simulink model "before_MPC"  (R2022b)
settings: Solver=VariableStepAuto  StartTime=0.0  StopTime=1e6  RelTol=1e-3
values from neighbouring files (symbols this model uses):
  BC = m/A/Cd    (= 136.363636364)    [ARES.m]    (also in control_before_MPC.m = 122; reference_signal_291123.m = 122; validation.m)
  Cd = 2.2    [ARES.m]    (also in control_before_MPC.m; control_script_291123.m; reference_signal_291123.m; validation.m)
  CL = Cd*E    (= 0)    [ARES.m]    (also in control_before_MPC.m; control_script_291123.m; reference_signal_291123.m; validation.m)
  F107_avg = 90.85    [ARES.m]    (also in control_before_MPC.m; control_script_291123.m; reference_signal_291123.m; validation.m)
  F107_day = 86.0    (= 86)    [ARES.m]    (also in control_before_MPC.m; control_script_291123.m; reference_signal_291123.m; validation.m)
  gamma0 = kepOut.gamma(end)    [ARES.m]    (also in control_before_MPC.m; control_script_291123.m; reference_signal_291123.m; validation.m)
  h0 = kepOut.h(end)    [ARES.m]    (also in control_before_MPC.m; control_script_291123.m; getSH.m = h0(n); reference_signal_291123.m)
  jdate = jdate+ndays1    [ARES.m]    (also in control_before_MPC.m; control_script_291123.m; reference_signal_291123.m; validation.m)
  Kp = 1    [ARES.m]    (also in control_before_MPC.m; control_script_291123.m; reference_signal_291123.m; validation.m)
  mi = 398600.44    [ARES.m]    (also in control_before_MPC.m; control_script_291123.m; reference_signal_291123.m; validation.m)
  r_a = alt_0+Re    (= 6771.0088)    [ARES.m]    (also in control_before_MPC.m = 6571.0088; control_script_291123.m = 6571.0088; reference_signal_291123.m = 6571.0088; validation.m = 6571.0088)
  Re = Re*1000    (= 6371008.8)    [ARES.m]    (also in control_before_MPC.m; control_script_291123.m; reference_signal_291123.m; trajectory_solver.m = 6378000)
  stop_h = 0    [ARES.m]    (also in control_before_MPC.m; control_script_291123.m; reference_signal_291123.m; validation.m)
  theta0 = kepOut.theta(end)    [ARES.m]    (also in control_before_MPC.m; control_script_291123.m; reference_signal_291123.m; validation.m)
  V0 = kepOut.V(end)    [ARES.m]    (also in control_before_MPC.m; control_script_291123.m; reference_signal_291123.m; validation.m)
  x0 = kepOut.x(end)    [ARES.m]    (also in control_before_MPC.m; control_script_291123.m; reference_signal_291123.m; validation.m)
libraries: simulink x2
settings Model: Creator=zhanghanwen  LastModifiedBy=zhanghanwen

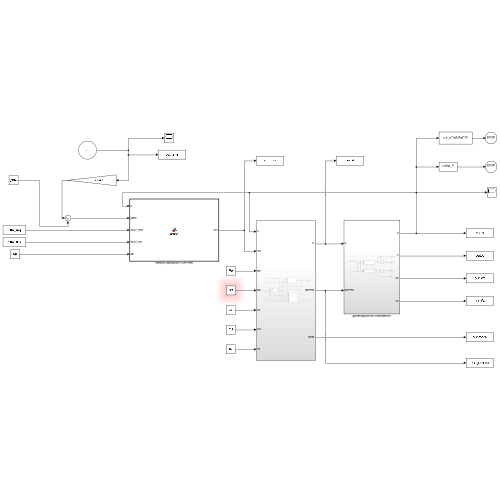
[thumbnail: Simulink's stored preview of the top-level diagram]
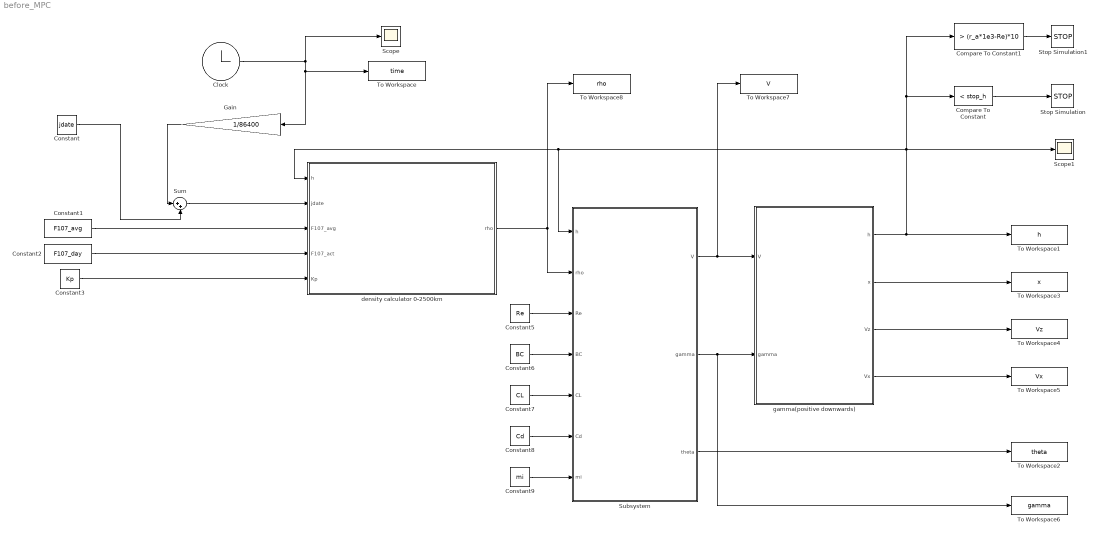
== system before_MPC ==
  Clock : Clock
  Compare To Constant : simulink/Logic and Bit Operations/Compare To Constant  relop=<  const=stop_h  OutDataTypeStr=boolean
  Compare To Constant1 : simulink/Logic and Bit Operations/Compare To Constant  relop=>  const=(r_a*1e3-Re)*10  OutDataTypeStr=boolean
  Constant : Constant  Value=jdate
  Constant1 : Constant  Value=F107_avg
  Constant2 : Constant  Value=F107_day
  Constant3 : Constant  Value=Kp
  Constant5 : Constant  Value=Re
  Constant6 : Constant  Value=BC
  Constant7 : Constant  Value=CL
  Constant8 : Constant  Value=Cd
  Constant9 : Constant  Value=mi
  Gain : Gain  Gain=1/86400
  Scope : Scope
  Scope1 : Scope
  Stop Simulation : Stop
  Stop Simulation1 : Stop
  Subsystem : Subsystem
  Sum : Sum  Inputs=|++
  To Workspace : ToWorkspace  VariableName=time  SampleTime=-1
      settings: Save2DSignal=2-D array (concatenate along first dimension)
  To Workspace1 : ToWorkspace  VariableName=h  SampleTime=-1
      settings: Save2DSignal=2-D array (concatenate along first dimension)
  To Workspace2 : ToWorkspace  VariableName=theta  SampleTime=-1
      settings: Save2DSignal=2-D array (concatenate along first dimension)
  To Workspace3 : ToWorkspace  VariableName=x  SampleTime=-1
  To Workspace4 : ToWorkspace  VariableName=Vz  SampleTime=-1
      settings: Save2DSignal=2-D array (concatenate along first dimension)
  To Workspace5 : ToWorkspace  VariableName=Vx  SampleTime=-1
      settings: Save2DSignal=2-D array (concatenate along first dimension)
  To Workspace6 : ToWorkspace  VariableName=gamma  SampleTime=-1
      settings: Save2DSignal=2-D array (concatenate along first dimension)
  To Workspace7 : ToWorkspace  VariableName=V  SampleTime=-1
      settings: Save2DSignal=2-D array (concatenate along first dimension)
  To Workspace8 : ToWorkspace  VariableName=rho  SampleTime=-1
      settings: Save2DSignal=2-D array (concatenate along first dimension)
  density calculator 0-2500km : MATLAB Function  TreatAsAtomicUnit=on
  gamma(positive downwards) : Subsystem
  wires:
  Clock/1 -> Gain/1, To Workspace/1, Scope/1
  Constant/1 -> Sum/2
  Sum/1 -> density calculator 0-2500km/2(jdate)
  Constant1/1 -> density calculator 0-2500km/3(F107_avg)
  Constant2/1 -> density calculator 0-2500km/4(F107_act)
  Constant3/1 -> density calculator 0-2500km/5(Kp)
  Gain/1 -> Sum/1
  density calculator 0-2500km/1(rho) -> To Workspace8/1, Subsystem/2(rho)
  Constant5/1 -> Subsystem/3(Re)
  Constant6/1 -> Subsystem/4(BC)
  Constant7/1 -> Subsystem/5(CL)
  Constant8/1 -> Subsystem/6(Cd)
  Constant9/1 -> Subsystem/7(mi)
  Subsystem/3(theta) -> To Workspace2/1
  Subsystem/2(gamma) -> To Workspace6/1, gamma(positive downwards)/2(gamma)
  Subsystem/1(V) -> To Workspace7/1, gamma(positive downwards)/1(V)
  gamma(positive downwards)/2(x) -> To Workspace3/1
  gamma(positive downwards)/3(Vz) -> To Workspace4/1
  gamma(positive downwards)/4(Vx) -> To Workspace5/1
  gamma(positive downwards)/1(h) -> Compare To Constant1/1, Compare To Constant/1, Subsystem/1(h), density calculator 0-2500km/1(h), Scope1/1, To Workspace1/1
  Compare To Constant/1 -> Stop Simulation/1
  Compare To Constant1/1 -> Stop Simulation1/1

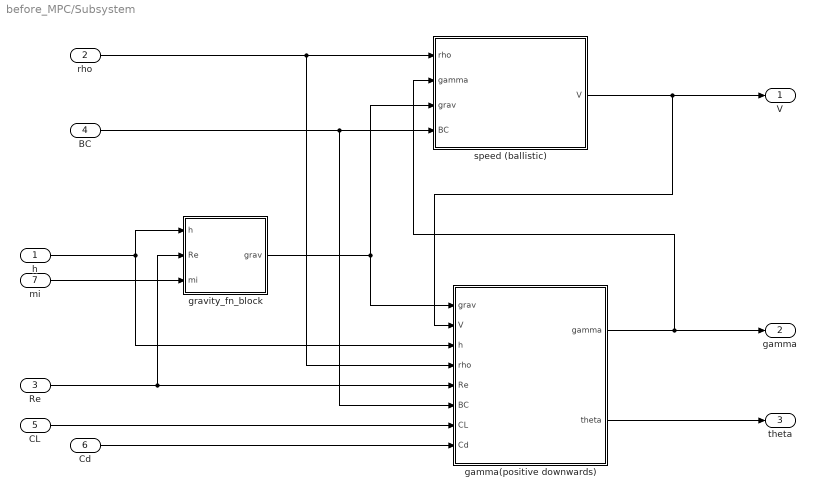
== system before_MPC/Subsystem ==
  h : Inport
  rho : Inport  Port=2
  Re : Inport  Port=3
  BC : Inport  Port=4
  CL : Inport  Port=5
  Cd : Inport  Port=6
  mi : Inport  Port=7
  gamma(positive downwards) : Subsystem
  gravity_fn_block : MATLAB Function  TreatAsAtomicUnit=on
  speed (ballistic) : Subsystem
  V : Outport
  gamma : Outport  Port=2
  theta : Outport  Port=3
  wires:
  rho/1 -> gamma(positive downwards)/4(rho), speed (ballistic)/1(rho)
  gravity_fn_block/1(grav) -> speed (ballistic)/3(grav), gamma(positive downwards)/1(grav)
  h/1 -> gravity_fn_block/1(h), gamma(positive downwards)/3(h)
  gamma(positive downwards)/1(gamma) -> speed (ballistic)/2(gamma), gamma/1
  gamma(positive downwards)/2(theta) -> theta/1
  speed (ballistic)/1(V) -> V/1, gamma(positive downwards)/2(V)
  Re/1 -> gravity_fn_block/2(Re), gamma(positive downwards)/5(Re)
  BC/1 -> gamma(positive downwards)/6(BC), speed (ballistic)/4(BC)
  CL/1 -> gamma(positive downwards)/7(CL)
  Cd/1 -> gamma(positive downwards)/8(Cd)
  mi/1 -> gravity_fn_block/3(mi)

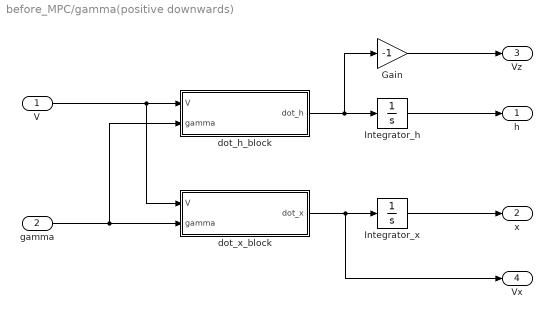
== system before_MPC/gamma(positive downwards) ==
  V : Inport
  gamma : Inport  Port=2
  Gain : Gain  Gain=-1
  Integrator_h : Integrator  InitialCondition=h0
  Integrator_x : Integrator  InitialCondition=x0
  dot_h_block : MATLAB Function  TreatAsAtomicUnit=on
  dot_x_block : MATLAB Function  TreatAsAtomicUnit=on
  h : Outport
  x : Outport  Port=2
  Vz : Outport  Port=3
  Vx : Outport  Port=4
  wires:
  V/1 -> dot_x_block/1(V), dot_h_block/1(V)
  gamma/1 -> dot_x_block/2(gamma), dot_h_block/2(gamma)
  Integrator_h/1 -> h/1
  dot_h_block/1(dot_h) -> Gain/1, Integrator_h/1
  Integrator_x/1 -> x/1
  dot_x_block/1(dot_x) -> Vx/1, Integrator_x/1
  Gain/1 -> Vz/1

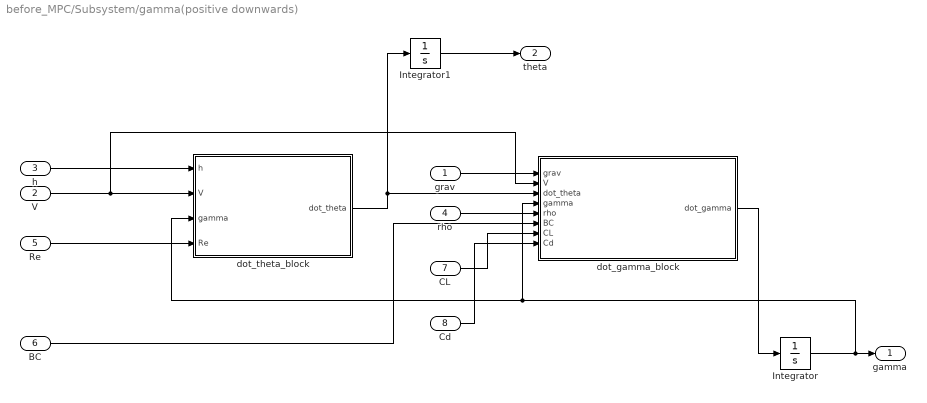
== system before_MPC/Subsystem/gamma(positive downwards) ==
  grav : Inport
  V : Inport  Port=2
  h : Inport  Port=3
  rho : Inport  Port=4
  Re : Inport  Port=5
  BC : Inport  Port=6
  CL : Inport  Port=7
  Cd : Inport  Port=8
  Integrator : Integrator  InitialCondition=gamma0  AbsoluteTolerance=1e-6  ZeroCross=off
  Integrator1 : Integrator  InitialCondition=theta0
  dot_gamma_block : MATLAB Function  TreatAsAtomicUnit=on
  dot_theta_block : MATLAB Function  TreatAsAtomicUnit=on
  gamma : Outport
  theta : Outport  Port=2
  wires:
  grav/1 -> dot_gamma_block/1(grav)
  dot_gamma_block/1(dot_gamma) -> Integrator/1
  dot_theta_block/1(dot_theta) -> Integrator1/1, dot_gamma_block/3(dot_theta)
  rho/1 -> dot_gamma_block/5(rho)
  h/1 -> dot_theta_block/1(h)
  V/1 -> dot_gamma_block/2(V), dot_theta_block/2(V)
  Integrator1/1 -> theta/1
  Integrator/1 -> dot_theta_block/3(gamma), dot_gamma_block/4(gamma), gamma/1
  Re/1 -> dot_theta_block/4(Re)
  BC/1 -> dot_gamma_block/6(BC)
  CL/1 -> dot_gamma_block/7(CL)
  Cd/1 -> dot_gamma_block/8(Cd)

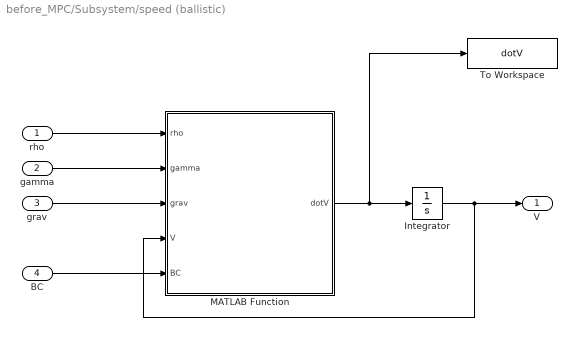
== system before_MPC/Subsystem/speed (ballistic) ==
  rho : Inport
  gamma : Inport  Port=2
  grav : Inport  Port=3
  BC : Inport  Port=4
  Integrator : Integrator  InitialCondition=V0
  MATLAB Function : MATLAB Function  TreatAsAtomicUnit=on
  To Workspace : ToWorkspace  VariableName=dotV  SampleTime=-1
      settings: Save2DSignal=2-D array (concatenate along first dimension)
  V : Outport
  wires:
  Integrator/1 -> MATLAB Function/4(V), V/1
  grav/1 -> MATLAB Function/3(grav)
  gamma/1 -> MATLAB Function/2(gamma)
  rho/1 -> MATLAB Function/1(rho)
  MATLAB Function/1(dotV) -> Integrator/1, To Workspace/1
  BC/1 -> MATLAB Function/5(BC)

== matlab function before_MPC/Subsystem/gravity_fn_block ==
  data: h input; grav output; Re input; mi input
function grav = gravity(h,Re,mi)

grav = mi*1e9 / (Re+h)^2;
end

== matlab function before_MPC/density calculator 0-2500km ==
  data: h input; jdate input; F107_avg input; rho output; F107_act input; Kp input
%This function combines Jacchia J71 and Exponential Atmosphere for %calculating density in the band [0;2500] km
%A transition function should be introduced to avoid discontinuities
function rho = unirho(h,jdate,F107_avg,F107_act,Kp) 
         h=h/1000; %conversion [m] to [km]
         rho = 1.225 * exp(- h/(8.3975));    % my Python model, using SH = 8.43 and rho0=1.221 as constant
    %from 0 to 100 km of altitude use Exponential Atmosphere
    % rho=0;
    % if h<100 && h>=0
    %    rho=expAtm(h);
    % end


    %A warning is printed if a negative altitude is predicted by %the simulation (due to Simulink discrete stopping criterion)
        if h<0
           % fprintf('Warning: mismatched density, altitude: %3.2e km',h) 
           rho=1.225;
        end
end




    
    %% Standard Density 
    
%This function calculates density through an exponential model
%rho=expAtm(H)
%H is the geopotential height in km
%rho is the density in kg/m^3
%rho0,h0,SH are updated each 10 km (source: Wertz, 1978)
% function rho=expAtm(H)
% [rho0,h0,SH]=getSH(H);
% rho=rho0*exp(-(H-h0)/SH);   %kg/m^3
% end

== matlab function before_MPC/Subsystem/speed (ballistic)/MATLAB Function ==
  data: rho input; dotV output; gamma input; grav input; V input; BC input
function dotV = dvdt(rho,gamma,grav,V,BC)
dotV = -0.5*rho*V^2/BC + grav*sin(gamma);
end

== matlab function before_MPC/Subsystem/gamma(positive downwards)/dot_theta_block ==
  data: h input; dot_theta output; V input; gamma input; Re input
function dot_theta = dthetadt(h,V,gamma,Re)


dot_theta = V*cos(gamma)/(Re+h); 

end

== matlab function before_MPC/Subsystem/gamma(positive downwards)/dot_gamma_block ==
  data: grav input; dot_gamma output; V input; dot_theta input; gamma input; rho input; BC input; CL input; Cd input
function dot_gamma = dgammadt(grav,V,dot_theta,gamma,rho,BC,CL,Cd)
dot_gamma = grav / V * cos(gamma) - dot_theta - 0.5 * rho/BC * CL / Cd*V; 
end

== matlab function before_MPC/gamma(positive downwards)/dot_h_block ==
  data: V input; dot_h output; gamma input
function dot_h = dhdt(V,gamma)
dot_h = -V*sin(gamma);
end

== matlab function before_MPC/gamma(positive downwards)/dot_x_block ==
  data: V input; dot_x output; gamma input
function dot_x = dxdt(V,gamma)
dot_x = -V*cos(gamma);
end
